simulink model "Events5"  (Simulink 6.0)
settings: Solver=FixedStepDiscrete  StartTime=0.0  StopTime=inf  RelTol=1e-3
settings Model: Creator=scaife  LastModifiedBy=scaife  ExtModeAutoUpdateStatusClock=off
settings DataIOCC: SignalLoggingName=sigsOut
settings DebuggingCC: AlgebraicLoopMsg=error  SolverPrmCheckMsg=none
settings HardwareCC: TargetUnknown=on
settings STFCustomTargetCC: TargetFcnLib=ansi_tfl_tmw.mat  GenFloatMathFcnCalls=ANSI_C  ModelReferenceCompliant=off  SystemTargetFile=grt.tlc

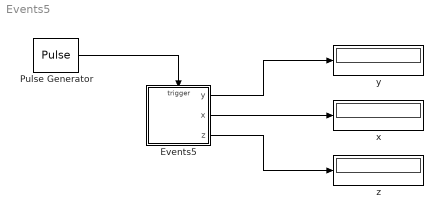
== system Events5 ==
  Events5 : Stateflow chart
  Pulse Generator : DiscretePulseGenerator
  x : Display
  y : Display
  z : Display
  wires:
  Pulse Generator/1 -> Events5/Trigger
  Events5/2(x) -> x/1
  Events5/3(z) -> z/1
  Events5/1(y) -> y/1

== stateflow chart Events5 ==
  state Top1 [parallel]
    state A/
      en: y++
    state D/
      en: y++
    state E/
      en: y++
    (default) -> A
    A -> D : E/send(F,B);z++
    D -> E : E/send(F,C);z++
    E -> A : E/F;z++
  state Top2 [parallel]
    state B/
      en: x++
    state C/
      en: x++
    (default) -> B
    B -> C : F
    C -> B : F
  data: y output double; x output double; z output double
  events: E input EITHER_EDGE_EVENT; F local EITHER_EDGE_EVENT
